simulink model "TST_InjCrv_PoI2AddCor"  (R2016b)
settings: Solver=FixedStepDiscrete  StartTime=0.0  StopTime=simTime  FixedStep=sampleTime  RelTol=1e-3
values from neighbouring files (symbols this model uses):
  testCase = 1    [initTST_InjCrv_PoI2AddCor_001.m]    (also in initTST_InjCrv_PoI2AddCor_002.m = 2; initTST_InjCrv_PoI2AddCor_003.m = 3; initTST_InjCrv_PoI2AddCor_004.m = 4)
libraries: simulink x29, UnitTest_Lib x24
(part 1 of 2)
settings Model: Creator=zhengjinyan  LastModifiedBy=zhengjinyan
settings DebuggingCC: SignalRangeChecking=error

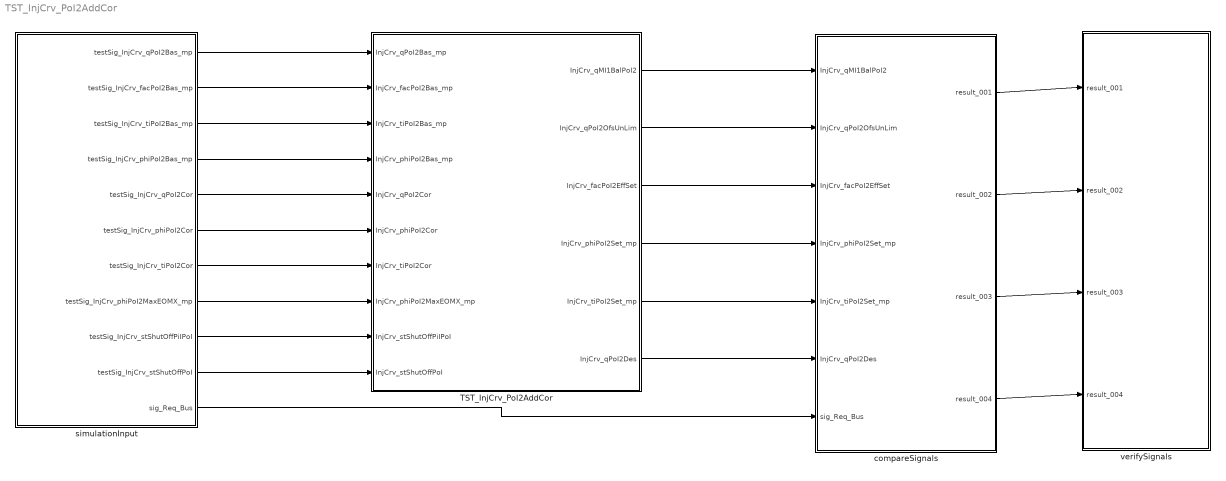
== system TST_InjCrv_PoI2AddCor ==
  TST_InjCrv_PoI2AddCor : Subsystem
  compareSignals : Subsystem
  simulationInput : Subsystem
  verifySignals : Subsystem
  wires:
  simulationInput/1(testSig_InjCrv_qPoI2Bas_mp) -> TST_InjCrv_PoI2AddCor/1(InjCrv_qPoI2Bas_mp)
  simulationInput/2(testSig_InjCrv_facPoI2Bas_mp) -> TST_InjCrv_PoI2AddCor/2(InjCrv_facPoI2Bas_mp)
  simulationInput/3(testSig_InjCrv_tiPoI2Bas_mp) -> TST_InjCrv_PoI2AddCor/3(InjCrv_tiPoI2Bas_mp)
  simulationInput/4(testSig_InjCrv_phiPoI2Bas_mp) -> TST_InjCrv_PoI2AddCor/4(InjCrv_phiPoI2Bas_mp)
  simulationInput/5(testSig_InjCrv_qPoI2Cor) -> TST_InjCrv_PoI2AddCor/5(InjCrv_qPoI2Cor)
  simulationInput/6(testSig_InjCrv_phiPoI2Cor) -> TST_InjCrv_PoI2AddCor/6(InjCrv_phiPoI2Cor)
  simulationInput/7(testSig_InjCrv_tiPoI2Cor) -> TST_InjCrv_PoI2AddCor/7(InjCrv_tiPoI2Cor)
  simulationInput/8(testSig_InjCrv_phiPoI2MaxEOMX_mp) -> TST_InjCrv_PoI2AddCor/8(InjCrv_phiPoI2MaxEOMX_mp)
  simulationInput/9(testSig_InjCrv_stShutOffPiIPoI) -> TST_InjCrv_PoI2AddCor/9(InjCrv_stShutOffPiIPoI)
  simulationInput/10(testSig_InjCrv_stShutOffPoI) -> TST_InjCrv_PoI2AddCor/10(InjCrv_stShutOffPoI)
  TST_InjCrv_PoI2AddCor/1(InjCrv_qMI1BalPoI2) -> compareSignals/1(InjCrv_qMI1BalPoI2)
  TST_InjCrv_PoI2AddCor/2(InjCrv_qPoI2OfsUnLim) -> compareSignals/2(InjCrv_qPoI2OfsUnLim)
  TST_InjCrv_PoI2AddCor/3(InjCrv_facPoI2EffSet) -> compareSignals/3(InjCrv_facPoI2EffSet)
  TST_InjCrv_PoI2AddCor/4(InjCrv_phiPoI2Set_mp) -> compareSignals/4(InjCrv_phiPoI2Set_mp)
  TST_InjCrv_PoI2AddCor/5(InjCrv_tiPoI2Set_mp) -> compareSignals/5(InjCrv_tiPoI2Set_mp)
  TST_InjCrv_PoI2AddCor/6(InjCrv_qPoI2Des) -> compareSignals/6(InjCrv_qPoI2Des)
  simulationInput/11(sig_Req_Bus) -> compareSignals/7(sig_Req_Bus)
  compareSignals/1(result_001) -> verifySignals/1(result_001)
  compareSignals/2(result_002) -> verifySignals/2(result_002)
  compareSignals/3(result_003) -> verifySignals/3(result_003)
  compareSignals/4(result_004) -> verifySignals/4(result_004)

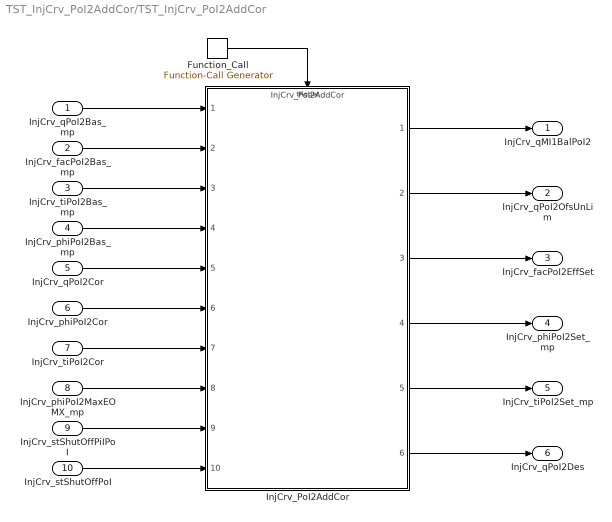
== system TST_InjCrv_PoI2AddCor/TST_InjCrv_PoI2AddCor ==
  InjCrv_qPoI2Bas_mp : Inport
  InjCrv_facPoI2Bas_mp : Inport  Port=2
  InjCrv_tiPoI2Bas_mp : Inport  Port=3
  InjCrv_phiPoI2Bas_mp : Inport  Port=4
  InjCrv_qPoI2Cor : Inport  Port=5
  InjCrv_phiPoI2Cor : Inport  Port=6
  InjCrv_tiPoI2Cor : Inport  Port=7
  InjCrv_phiPoI2MaxEOMX_mp : Inport  Port=8
  InjCrv_stShutOffPiIPoI : Inport  Port=9
  InjCrv_stShutOffPoI : Inport  Port=10
  Function_Call : simulink/Ports & Subsystems/Function-Call Generator  sample_time=sampleTime  numberOfIterations=1
  InjCrv_PoI2AddCor : ModelReference  ModelNameDialog=InjCrv_PoI2AddCor  SimulationMode=Normal  ModelReferenceVersion=1.19  TriggerPortName=function  TriggerPortTriggerType=function-call  TriggerPortStatesWhenEnabling=held
  InjCrv_qMI1BalPoI2 : Outport
  InjCrv_qPoI2OfsUnLim : Outport  Port=2
  InjCrv_facPoI2EffSet : Outport  Port=3
  InjCrv_phiPoI2Set_mp : Outport  Port=4
  InjCrv_tiPoI2Set_mp : Outport  Port=5
  InjCrv_qPoI2Des : Outport  Port=6
  wires:
  Function_Call/1 -> InjCrv_PoI2AddCor/Trigger
  InjCrv_qPoI2Bas_mp/1 -> InjCrv_PoI2AddCor/1
  InjCrv_facPoI2Bas_mp/1 -> InjCrv_PoI2AddCor/2
  InjCrv_tiPoI2Bas_mp/1 -> InjCrv_PoI2AddCor/3
  InjCrv_phiPoI2Bas_mp/1 -> InjCrv_PoI2AddCor/4
  InjCrv_qPoI2Cor/1 -> InjCrv_PoI2AddCor/5
  InjCrv_phiPoI2Cor/1 -> InjCrv_PoI2AddCor/6
  InjCrv_tiPoI2Cor/1 -> InjCrv_PoI2AddCor/7
  InjCrv_phiPoI2MaxEOMX_mp/1 -> InjCrv_PoI2AddCor/8
  InjCrv_stShutOffPiIPoI/1 -> InjCrv_PoI2AddCor/9
  InjCrv_stShutOffPoI/1 -> InjCrv_PoI2AddCor/10
  InjCrv_PoI2AddCor/1 -> InjCrv_qMI1BalPoI2/1
  InjCrv_PoI2AddCor/2 -> InjCrv_qPoI2OfsUnLim/1
  InjCrv_PoI2AddCor/3 -> InjCrv_facPoI2EffSet/1
  InjCrv_PoI2AddCor/4 -> InjCrv_phiPoI2Set_mp/1
  InjCrv_PoI2AddCor/5 -> InjCrv_tiPoI2Set_mp/1
  InjCrv_PoI2AddCor/6 -> InjCrv_qPoI2Des/1

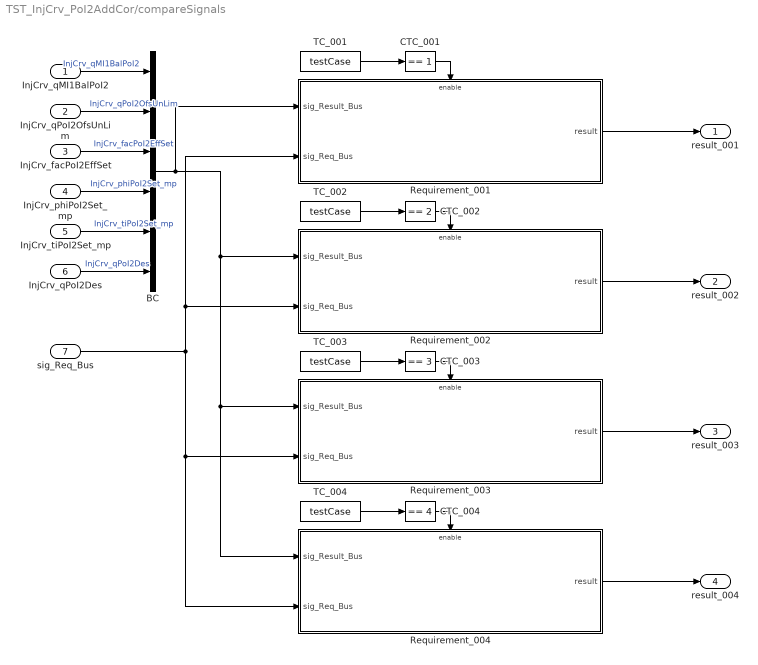
== system TST_InjCrv_PoI2AddCor/compareSignals ==
  InjCrv_qMI1BalPoI2 : Inport
  InjCrv_qPoI2OfsUnLim : Inport  Port=2
  InjCrv_facPoI2EffSet : Inport  Port=3
  InjCrv_phiPoI2Set_mp : Inport  Port=4
  InjCrv_tiPoI2Set_mp : Inport  Port=5
  InjCrv_qPoI2Des : Inport  Port=6
  sig_Req_Bus : Inport  Port=7
  BC : BusCreator  Inputs=6
  CTC_001 : simulink/Logic and Bit Operations/Compare To Constant  relop===  const=1  OutDataTypeStr=boolean
  CTC_002 : simulink/Logic and Bit Operations/Compare To Constant  relop===  const=2  OutDataTypeStr=boolean
  CTC_003 : simulink/Logic and Bit Operations/Compare To Constant  relop===  const=3  OutDataTypeStr=boolean
  CTC_004 : simulink/Logic and Bit Operations/Compare To Constant  relop===  const=4  OutDataTypeStr=boolean
  Requirement_001 : Subsystem
  Requirement_002 : Subsystem
  Requirement_003 : Subsystem
  Requirement_004 : Subsystem
  TC_001 : Constant  Value=testCase
  TC_002 : Constant  Value=testCase
  TC_003 : Constant  Value=testCase
  TC_004 : Constant  Value=testCase
  result_001 : Outport
  result_002 : Outport  Port=2
  result_003 : Outport  Port=3
  result_004 : Outport  Port=4
  wires:
  InjCrv_qMI1BalPoI2/1 -> BC/1  "InjCrv_qMI1BalPoI2"
  InjCrv_qPoI2OfsUnLim/1 -> BC/2  "InjCrv_qPoI2OfsUnLim"
  InjCrv_facPoI2EffSet/1 -> BC/3  "InjCrv_facPoI2EffSet"
  InjCrv_phiPoI2Set_mp/1 -> BC/4  "InjCrv_phiPoI2Set_mp"
  InjCrv_tiPoI2Set_mp/1 -> BC/5  "InjCrv_tiPoI2Set_mp"
  InjCrv_qPoI2Des/1 -> BC/6  "InjCrv_qPoI2Des"
  TC_001/1 -> CTC_001/1
  CTC_001/1 -> Requirement_001/Enable
  sig_Req_Bus/1 -> Requirement_003/2(sig_Req_Bus), Requirement_004/2(sig_Req_Bus), Requirement_001/2(sig_Req_Bus), Requirement_002/2(sig_Req_Bus)
  BC/1 -> Requirement_003/1(sig_Result_Bus), Requirement_004/1(sig_Result_Bus), Requirement_002/1(sig_Result_Bus), Requirement_001/1(sig_Result_Bus)
  Requirement_001/1(result) -> result_001/1
  TC_002/1 -> CTC_002/1
  CTC_002/1 -> Requirement_002/Enable
  Requirement_002/1(result) -> result_002/1
  TC_003/1 -> CTC_003/1
  CTC_003/1 -> Requirement_003/Enable
  Requirement_003/1(result) -> result_003/1
  TC_004/1 -> CTC_004/1
  CTC_004/1 -> Requirement_004/Enable
  Requirement_004/1(result) -> result_004/1

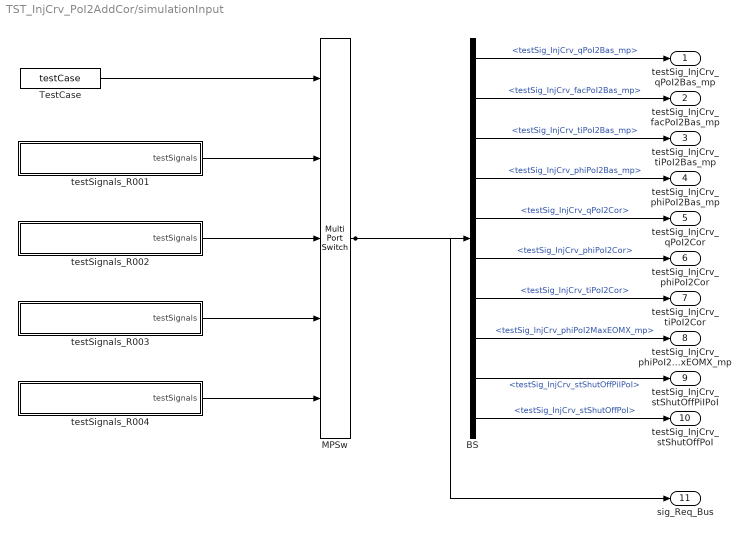
== system TST_InjCrv_PoI2AddCor/simulationInput ==
  BS : BusSelector  OutputSignals=testSig_InjCrv_qPoI2Bas_mp,testSig_InjCrv_facPoI2Bas_mp,testSig_InjCrv_tiPoI2Bas_mp,testSig_InjCrv_phiPoI2Bas_mp,testSig_InjCrv_qPoI2Cor,testSig_InjCrv_phiPoI2Cor,testSig_InjCrv_tiPoI2Cor,testSig_InjCrv_phiPoI2MaxEOMX_mp,testSig_InjCrv_stShutOffPiIPoI,testSig_InjCrv_stShutOffPoI
  MPSw : MultiPortSwitch  Inputs=4  SaturateOnIntegerOverflow=on  InputSameDT=on
  TestCase : Constant  Value=testCase
  testSignals_R001 : Subsystem
  testSignals_R002 : Subsystem
  testSignals_R003 : Subsystem
  testSignals_R004 : Subsystem
  testSig_InjCrv_qPoI2Bas_mp : Outport
  testSig_InjCrv_facPoI2Bas_mp : Outport  Port=2
  testSig_InjCrv_tiPoI2Bas_mp : Outport  Port=3
  testSig_InjCrv_phiPoI2Bas_mp : Outport  Port=4
  testSig_InjCrv_qPoI2Cor : Outport  Port=5
  testSig_InjCrv_phiPoI2Cor : Outport  Port=6
  testSig_InjCrv_tiPoI2Cor : Outport  Port=7
  testSig_InjCrv_phiPoI2MaxEOMX_mp : Outport  Port=8
  testSig_InjCrv_stShutOffPiIPoI : Outport  Port=9
  testSig_InjCrv_stShutOffPoI : Outport  Port=10
  sig_Req_Bus : Outport  Port=11
  wires:
  BS/1 -> testSig_InjCrv_qPoI2Bas_mp/1  "<testSig_InjCrv_qPoI2Bas_mp>"
  BS/2 -> testSig_InjCrv_facPoI2Bas_mp/1  "<testSig_InjCrv_facPoI2Bas_mp>"
  BS/3 -> testSig_InjCrv_tiPoI2Bas_mp/1  "<testSig_InjCrv_tiPoI2Bas_mp>"
  BS/4 -> testSig_InjCrv_phiPoI2Bas_mp/1  "<testSig_InjCrv_phiPoI2Bas_mp>"
  BS/5 -> testSig_InjCrv_qPoI2Cor/1  "<testSig_InjCrv_qPoI2Cor>"
  BS/6 -> testSig_InjCrv_phiPoI2Cor/1  "<testSig_InjCrv_phiPoI2Cor>"
  BS/7 -> testSig_InjCrv_tiPoI2Cor/1  "<testSig_InjCrv_tiPoI2Cor>"
  BS/8 -> testSig_InjCrv_phiPoI2MaxEOMX_mp/1  "<testSig_InjCrv_phiPoI2MaxEOMX_mp>"
  BS/9 -> testSig_InjCrv_stShutOffPiIPoI/1  "<testSig_InjCrv_stShutOffPiIPoI>"
  BS/10 -> testSig_InjCrv_stShutOffPoI/1  "<testSig_InjCrv_stShutOffPoI>"
  MPSw/1 -> BS/1, sig_Req_Bus/1
  TestCase/1 -> MPSw/1
  testSignals_R001/1(testSignals) -> MPSw/2
  testSignals_R002/1(testSignals) -> MPSw/3
  testSignals_R003/1(testSignals) -> MPSw/4
  testSignals_R004/1(testSignals) -> MPSw/5

== system TST_InjCrv_PoI2AddCor/verifySignals ==
  result_001 : Inport
  result_002 : Inport  Port=2
  result_003 : Inport  Port=3
  result_004 : Inport  Port=4
  Assertion_001 : Assertion  Enabled=off
  Assertion_002 : Assertion  Enabled=off
  Assertion_003 : Assertion  Enabled=off
  Assertion_004 : Assertion  Enabled=off
  wires:
  result_001/1 -> Assertion_001/1
  result_002/1 -> Assertion_002/1
  result_003/1 -> Assertion_003/1
  result_004/1 -> Assertion_004/1

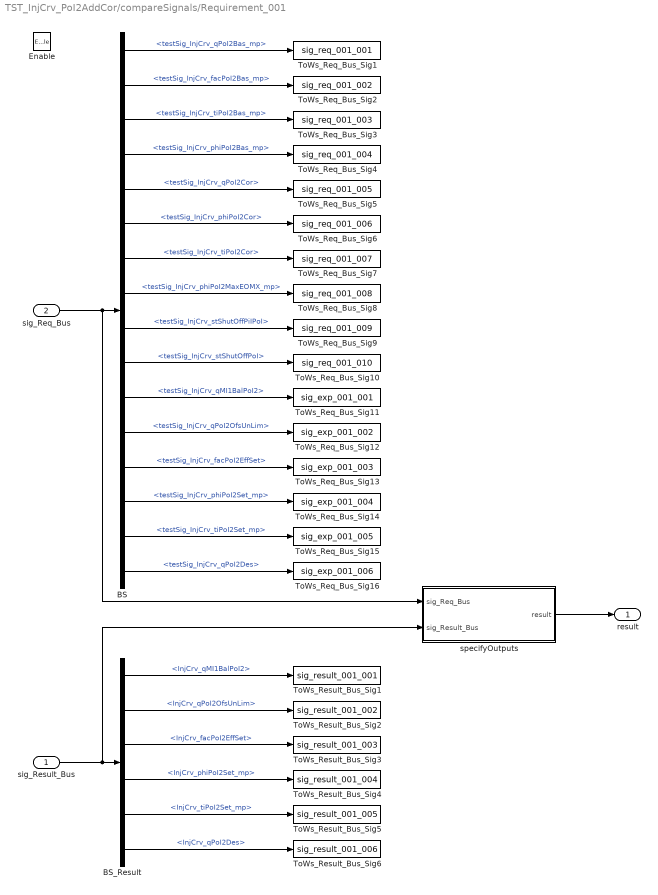
== system TST_InjCrv_PoI2AddCor/compareSignals/Requirement_001 ==
  sig_Result_Bus : Inport
  sig_Req_Bus : Inport  Port=2
  Enable : EnablePort
  BS : BusSelector  OutputSignals=testSig_InjCrv_qPoI2Bas_mp,testSig_InjCrv_facPoI2Bas_mp,testSig_InjCrv_tiPoI2Bas_mp,testSig_InjCrv_phiPoI2Bas_mp,testSig_InjCrv_qPoI2Cor,testSig_InjCrv_phiPoI2Cor,testSig_InjCrv_tiPoI2Cor,testSig_InjCrv_phiPoI2MaxEOMX_mp,testSig_InjCrv_stShutOffPiIPoI,testSig_InjCrv_stShutOffPoI,testSig_InjCrv_qMI1BalPoI2,testSig_InjCrv_qPoI2OfsUnLim,testSig_InjCrv_facPoI2EffSet,testSig_InjCrv_phiPoI2Set_mp,testSig_InjCrv_tiPoI2Set_mp,testSig_InjCrv_qPoI2Des
  BS_Result : BusSelector  OutputSignals=InjCrv_qMI1BalPoI2,InjCrv_qPoI2OfsUnLim,InjCrv_facPoI2EffSet,InjCrv_phiPoI2Set_mp,InjCrv_tiPoI2Set_mp,InjCrv_qPoI2Des
  ToWs_Req_Bus_Sig1 : ToWorkspace  VariableName=sig_req_001_001  SaveFormat=Structure With Time
  ToWs_Req_Bus_Sig10 : ToWorkspace  VariableName=sig_req_001_010  SaveFormat=Structure With Time
  ToWs_Req_Bus_Sig11 : ToWorkspace  VariableName=sig_exp_001_001  SaveFormat=Structure With Time
  ToWs_Req_Bus_Sig12 : ToWorkspace  VariableName=sig_exp_001_002  SaveFormat=Structure With Time
  ToWs_Req_Bus_Sig13 : ToWorkspace  VariableName=sig_exp_001_003  SaveFormat=Structure With Time
  ToWs_Req_Bus_Sig14 : ToWorkspace  VariableName=sig_exp_001_004  SaveFormat=Structure With Time
  ToWs_Req_Bus_Sig15 : ToWorkspace  VariableName=sig_exp_001_005  SaveFormat=Structure With Time
  ToWs_Req_Bus_Sig16 : ToWorkspace  VariableName=sig_exp_001_006  SaveFormat=Structure With Time
  ToWs_Req_Bus_Sig2 : ToWorkspace  VariableName=sig_req_001_002  SaveFormat=Structure With Time
  ToWs_Req_Bus_Sig3 : ToWorkspace  VariableName=sig_req_001_003  SaveFormat=Structure With Time
  ToWs_Req_Bus_Sig4 : ToWorkspace  VariableName=sig_req_001_004  SaveFormat=Structure With Time
  ToWs_Req_Bus_Sig5 : ToWorkspace  VariableName=sig_req_001_005  SaveFormat=Structure With Time
  ToWs_Req_Bus_Sig6 : ToWorkspace  VariableName=sig_req_001_006  SaveFormat=Structure With Time
  ToWs_Req_Bus_Sig7 : ToWorkspace  VariableName=sig_req_001_007  SaveFormat=Structure With Time
  ToWs_Req_Bus_Sig8 : ToWorkspace  VariableName=sig_req_001_008  SaveFormat=Structure With Time
  ToWs_Req_Bus_Sig9 : ToWorkspace  VariableName=sig_req_001_009  SaveFormat=Structure With Time
  ToWs_Result_Bus_Sig1 : ToWorkspace  VariableName=sig_result_001_001  SaveFormat=Structure With Time
  ToWs_Result_Bus_Sig2 : ToWorkspace  VariableName=sig_result_001_002  SaveFormat=Structure With Time
  ToWs_Result_Bus_Sig3 : ToWorkspace  VariableName=sig_result_001_003  SaveFormat=Structure With Time
  ToWs_Result_Bus_Sig4 : ToWorkspace  VariableName=sig_result_001_004  SaveFormat=Structure With Time
  ToWs_Result_Bus_Sig5 : ToWorkspace  VariableName=sig_result_001_005  SaveFormat=Structure With Time
  ToWs_Result_Bus_Sig6 : ToWorkspace  VariableName=sig_result_001_006  SaveFormat=Structure With Time
  specifyOutputs : Subsystem
  result : Outport
  wires:
  sig_Req_Bus/1 -> BS/1, specifyOutputs/1(sig_Req_Bus)
  BS/1 -> ToWs_Req_Bus_Sig1/1  "<testSig_InjCrv_qPoI2Bas_mp>"
  BS/2 -> ToWs_Req_Bus_Sig2/1  "<testSig_InjCrv_facPoI2Bas_mp>"
  BS/3 -> ToWs_Req_Bus_Sig3/1  "<testSig_InjCrv_tiPoI2Bas_mp>"
  BS/4 -> ToWs_Req_Bus_Sig4/1  "<testSig_InjCrv_phiPoI2Bas_mp>"
  BS/5 -> ToWs_Req_Bus_Sig5/1  "<testSig_InjCrv_qPoI2Cor>"
  BS/6 -> ToWs_Req_Bus_Sig6/1  "<testSig_InjCrv_phiPoI2Cor>"
  BS/7 -> ToWs_Req_Bus_Sig7/1  "<testSig_InjCrv_tiPoI2Cor>"
  BS/8 -> ToWs_Req_Bus_Sig8/1  "<testSig_InjCrv_phiPoI2MaxEOMX_mp>"
  BS/9 -> ToWs_Req_Bus_Sig9/1  "<testSig_InjCrv_stShutOffPiIPoI>"
  BS/10 -> ToWs_Req_Bus_Sig10/1  "<testSig_InjCrv_stShutOffPoI>"
  BS/11 -> ToWs_Req_Bus_Sig11/1  "<testSig_InjCrv_qMI1BalPoI2>"
  BS/12 -> ToWs_Req_Bus_Sig12/1  "<testSig_InjCrv_qPoI2OfsUnLim>"
  BS/13 -> ToWs_Req_Bus_Sig13/1  "<testSig_InjCrv_facPoI2EffSet>"
  BS/14 -> ToWs_Req_Bus_Sig14/1  "<testSig_InjCrv_phiPoI2Set_mp>"
  BS/15 -> ToWs_Req_Bus_Sig15/1  "<testSig_InjCrv_tiPoI2Set_mp>"
  BS/16 -> ToWs_Req_Bus_Sig16/1  "<testSig_InjCrv_qPoI2Des>"
  sig_Result_Bus/1 -> BS_Result/1, specifyOutputs/2(sig_Result_Bus)
  BS_Result/1 -> ToWs_Result_Bus_Sig1/1  "<InjCrv_qMI1BalPoI2>"
  BS_Result/2 -> ToWs_Result_Bus_Sig2/1  "<InjCrv_qPoI2OfsUnLim>"
  BS_Result/3 -> ToWs_Result_Bus_Sig3/1  "<InjCrv_facPoI2EffSet>"
  BS_Result/4 -> ToWs_Result_Bus_Sig4/1  "<InjCrv_phiPoI2Set_mp>"
  BS_Result/5 -> ToWs_Result_Bus_Sig5/1  "<InjCrv_tiPoI2Set_mp>"
  BS_Result/6 -> ToWs_Result_Bus_Sig6/1  "<InjCrv_qPoI2Des>"
  specifyOutputs/1(result) -> result/1

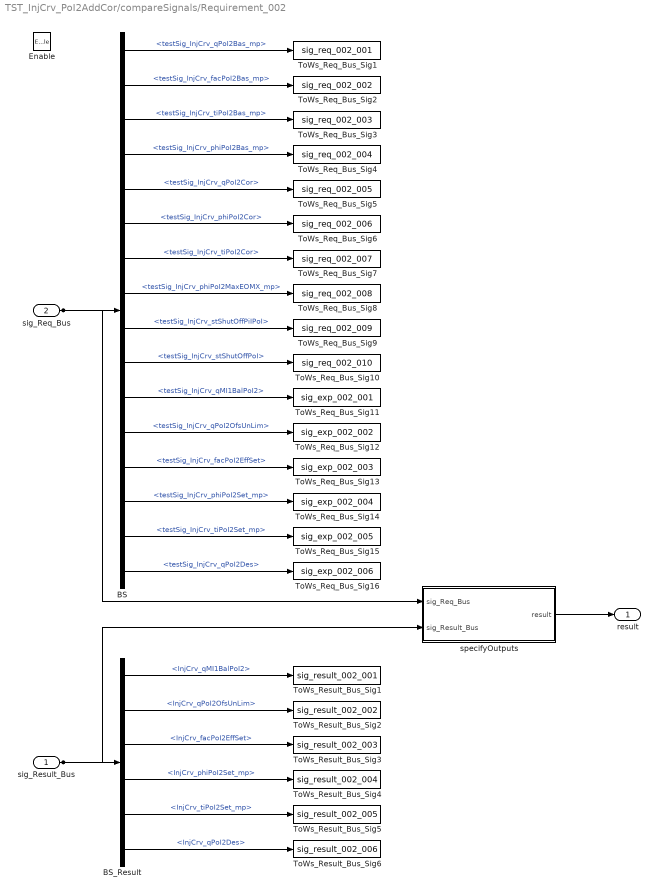
== system TST_InjCrv_PoI2AddCor/compareSignals/Requirement_002 ==
  sig_Result_Bus : Inport
  sig_Req_Bus : Inport  Port=2
  Enable : EnablePort
  BS : BusSelector  OutputSignals=testSig_InjCrv_qPoI2Bas_mp,testSig_InjCrv_facPoI2Bas_mp,testSig_InjCrv_tiPoI2Bas_mp,testSig_InjCrv_phiPoI2Bas_mp,testSig_InjCrv_qPoI2Cor,testSig_InjCrv_phiPoI2Cor,testSig_InjCrv_tiPoI2Cor,testSig_InjCrv_phiPoI2MaxEOMX_mp,testSig_InjCrv_stShutOffPiIPoI,testSig_InjCrv_stShutOffPoI,testSig_InjCrv_qMI1BalPoI2,testSig_InjCrv_qPoI2OfsUnLim,testSig_InjCrv_facPoI2EffSet,testSig_InjCrv_phiPoI2Set_mp,testSig_InjCrv_tiPoI2Set_mp,testSig_InjCrv_qPoI2Des
  BS_Result : BusSelector  OutputSignals=InjCrv_qMI1BalPoI2,InjCrv_qPoI2OfsUnLim,InjCrv_facPoI2EffSet,InjCrv_phiPoI2Set_mp,InjCrv_tiPoI2Set_mp,InjCrv_qPoI2Des
  ToWs_Req_Bus_Sig1 : ToWorkspace  VariableName=sig_req_002_001  SaveFormat=Structure With Time
  ToWs_Req_Bus_Sig10 : ToWorkspace  VariableName=sig_req_002_010  SaveFormat=Structure With Time
  ToWs_Req_Bus_Sig11 : ToWorkspace  VariableName=sig_exp_002_001  SaveFormat=Structure With Time
  ToWs_Req_Bus_Sig12 : ToWorkspace  VariableName=sig_exp_002_002  SaveFormat=Structure With Time
  ToWs_Req_Bus_Sig13 : ToWorkspace  VariableName=sig_exp_002_003  SaveFormat=Structure With Time
  ToWs_Req_Bus_Sig14 : ToWorkspace  VariableName=sig_exp_002_004  SaveFormat=Structure With Time
  ToWs_Req_Bus_Sig15 : ToWorkspace  VariableName=sig_exp_002_005  SaveFormat=Structure With Time
  ToWs_Req_Bus_Sig16 : ToWorkspace  VariableName=sig_exp_002_006  SaveFormat=Structure With Time
  ToWs_Req_Bus_Sig2 : ToWorkspace  VariableName=sig_req_002_002  SaveFormat=Structure With Time
  ToWs_Req_Bus_Sig3 : ToWorkspace  VariableName=sig_req_002_003  SaveFormat=Structure With Time
  ToWs_Req_Bus_Sig4 : ToWorkspace  VariableName=sig_req_002_004  SaveFormat=Structure With Time
  ToWs_Req_Bus_Sig5 : ToWorkspace  VariableName=sig_req_002_005  SaveFormat=Structure With Time
  ToWs_Req_Bus_Sig6 : ToWorkspace  VariableName=sig_req_002_006  SaveFormat=Structure With Time
  ToWs_Req_Bus_Sig7 : ToWorkspace  VariableName=sig_req_002_007  SaveFormat=Structure With Time
  ToWs_Req_Bus_Sig8 : ToWorkspace  VariableName=sig_req_002_008  SaveFormat=Structure With Time
  ToWs_Req_Bus_Sig9 : ToWorkspace  VariableName=sig_req_002_009  SaveFormat=Structure With Time
  ToWs_Result_Bus_Sig1 : ToWorkspace  VariableName=sig_result_002_001  SaveFormat=Structure With Time
  ToWs_Result_Bus_Sig2 : ToWorkspace  VariableName=sig_result_002_002  SaveFormat=Structure With Time
  ToWs_Result_Bus_Sig3 : ToWorkspace  VariableName=sig_result_002_003  SaveFormat=Structure With Time
  ToWs_Result_Bus_Sig4 : ToWorkspace  VariableName=sig_result_002_004  SaveFormat=Structure With Time
  ToWs_Result_Bus_Sig5 : ToWorkspace  VariableName=sig_result_002_005  SaveFormat=Structure With Time
  ToWs_Result_Bus_Sig6 : ToWorkspace  VariableName=sig_result_002_006  SaveFormat=Structure With Time
  specifyOutputs : Subsystem
  result : Outport
  wires:
  sig_Req_Bus/1 -> BS/1, specifyOutputs/1(sig_Req_Bus)
  BS/1 -> ToWs_Req_Bus_Sig1/1  "<testSig_InjCrv_qPoI2Bas_mp>"
  BS/2 -> ToWs_Req_Bus_Sig2/1  "<testSig_InjCrv_facPoI2Bas_mp>"
  BS/3 -> ToWs_Req_Bus_Sig3/1  "<testSig_InjCrv_tiPoI2Bas_mp>"
  BS/4 -> ToWs_Req_Bus_Sig4/1  "<testSig_InjCrv_phiPoI2Bas_mp>"
  BS/5 -> ToWs_Req_Bus_Sig5/1  "<testSig_InjCrv_qPoI2Cor>"
  BS/6 -> ToWs_Req_Bus_Sig6/1  "<testSig_InjCrv_phiPoI2Cor>"
  BS/7 -> ToWs_Req_Bus_Sig7/1  "<testSig_InjCrv_tiPoI2Cor>"
  BS/8 -> ToWs_Req_Bus_Sig8/1  "<testSig_InjCrv_phiPoI2MaxEOMX_mp>"
  BS/9 -> ToWs_Req_Bus_Sig9/1  "<testSig_InjCrv_stShutOffPiIPoI>"
  BS/10 -> ToWs_Req_Bus_Sig10/1  "<testSig_InjCrv_stShutOffPoI>"
  BS/11 -> ToWs_Req_Bus_Sig11/1  "<testSig_InjCrv_qMI1BalPoI2>"
  BS/12 -> ToWs_Req_Bus_Sig12/1  "<testSig_InjCrv_qPoI2OfsUnLim>"
  BS/13 -> ToWs_Req_Bus_Sig13/1  "<testSig_InjCrv_facPoI2EffSet>"
  BS/14 -> ToWs_Req_Bus_Sig14/1  "<testSig_InjCrv_phiPoI2Set_mp>"
  BS/15 -> ToWs_Req_Bus_Sig15/1  "<testSig_InjCrv_tiPoI2Set_mp>"
  BS/16 -> ToWs_Req_Bus_Sig16/1  "<testSig_InjCrv_qPoI2Des>"
  sig_Result_Bus/1 -> BS_Result/1, specifyOutputs/2(sig_Result_Bus)
  BS_Result/1 -> ToWs_Result_Bus_Sig1/1  "<InjCrv_qMI1BalPoI2>"
  BS_Result/2 -> ToWs_Result_Bus_Sig2/1  "<InjCrv_qPoI2OfsUnLim>"
  BS_Result/3 -> ToWs_Result_Bus_Sig3/1  "<InjCrv_facPoI2EffSet>"
  BS_Result/4 -> ToWs_Result_Bus_Sig4/1  "<InjCrv_phiPoI2Set_mp>"
  BS_Result/5 -> ToWs_Result_Bus_Sig5/1  "<InjCrv_tiPoI2Set_mp>"
  BS_Result/6 -> ToWs_Result_Bus_Sig6/1  "<InjCrv_qPoI2Des>"
  specifyOutputs/1(result) -> result/1

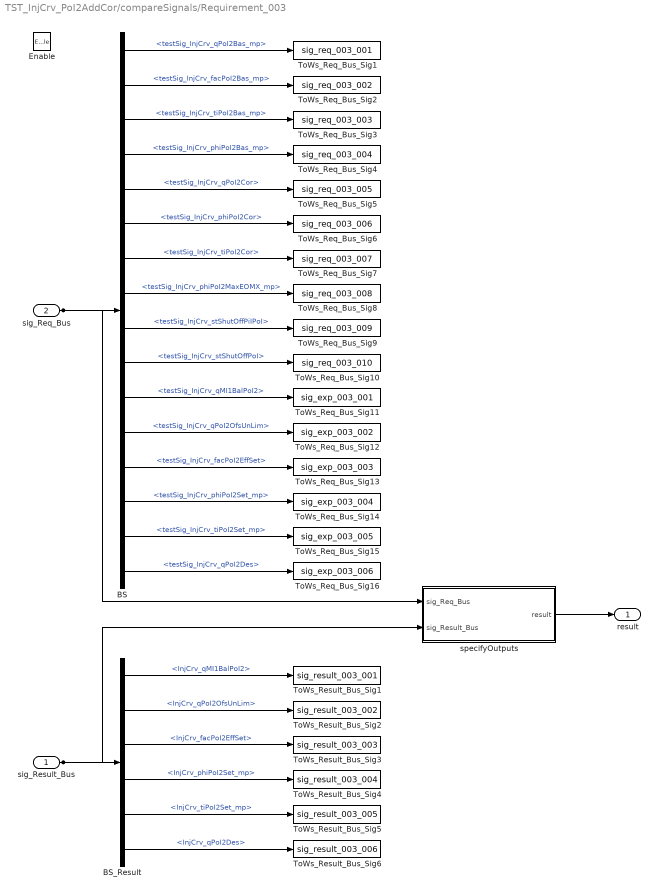
== system TST_InjCrv_PoI2AddCor/compareSignals/Requirement_003 ==
  sig_Result_Bus : Inport
  sig_Req_Bus : Inport  Port=2
  Enable : EnablePort
  BS : BusSelector  OutputSignals=testSig_InjCrv_qPoI2Bas_mp,testSig_InjCrv_facPoI2Bas_mp,testSig_InjCrv_tiPoI2Bas_mp,testSig_InjCrv_phiPoI2Bas_mp,testSig_InjCrv_qPoI2Cor,testSig_InjCrv_phiPoI2Cor,testSig_InjCrv_tiPoI2Cor,testSig_InjCrv_phiPoI2MaxEOMX_mp,testSig_InjCrv_stShutOffPiIPoI,testSig_InjCrv_stShutOffPoI,testSig_InjCrv_qMI1BalPoI2,testSig_InjCrv_qPoI2OfsUnLim,testSig_InjCrv_facPoI2EffSet,testSig_InjCrv_phiPoI2Set_mp,testSig_InjCrv_tiPoI2Set_mp,testSig_InjCrv_qPoI2Des
  BS_Result : BusSelector  OutputSignals=InjCrv_qMI1BalPoI2,InjCrv_qPoI2OfsUnLim,InjCrv_facPoI2EffSet,InjCrv_phiPoI2Set_mp,InjCrv_tiPoI2Set_mp,InjCrv_qPoI2Des
  ToWs_Req_Bus_Sig1 : ToWorkspace  VariableName=sig_req_003_001  SaveFormat=Structure With Time
  ToWs_Req_Bus_Sig10 : ToWorkspace  VariableName=sig_req_003_010  SaveFormat=Structure With Time
  ToWs_Req_Bus_Sig11 : ToWorkspace  VariableName=sig_exp_003_001  SaveFormat=Structure With Time
  ToWs_Req_Bus_Sig12 : ToWorkspace  VariableName=sig_exp_003_002  SaveFormat=Structure With Time
  ToWs_Req_Bus_Sig13 : ToWorkspace  VariableName=sig_exp_003_003  SaveFormat=Structure With Time
  ToWs_Req_Bus_Sig14 : ToWorkspace  VariableName=sig_exp_003_004  SaveFormat=Structure With Time
  ToWs_Req_Bus_Sig15 : ToWorkspace  VariableName=sig_exp_003_005  SaveFormat=Structure With Time
  ToWs_Req_Bus_Sig16 : ToWorkspace  VariableName=sig_exp_003_006  SaveFormat=Structure With Time
  ToWs_Req_Bus_Sig2 : ToWorkspace  VariableName=sig_req_003_002  SaveFormat=Structure With Time
  ToWs_Req_Bus_Sig3 : ToWorkspace  VariableName=sig_req_003_003  SaveFormat=Structure With Time
  ToWs_Req_Bus_Sig4 : ToWorkspace  VariableName=sig_req_003_004  SaveFormat=Structure With Time
  ToWs_Req_Bus_Sig5 : ToWorkspace  VariableName=sig_req_003_005  SaveFormat=Structure With Time
  ToWs_Req_Bus_Sig6 : ToWorkspace  VariableName=sig_req_003_006  SaveFormat=Structure With Time
  ToWs_Req_Bus_Sig7 : ToWorkspace  VariableName=sig_req_003_007  SaveFormat=Structure With Time
  ToWs_Req_Bus_Sig8 : ToWorkspace  VariableName=sig_req_003_008  SaveFormat=Structure With Time
  ToWs_Req_Bus_Sig9 : ToWorkspace  VariableName=sig_req_003_009  SaveFormat=Structure With Time
  ToWs_Result_Bus_Sig1 : ToWorkspace  VariableName=sig_result_003_001  SaveFormat=Structure With Time
  ToWs_Result_Bus_Sig2 : ToWorkspace  VariableName=sig_result_003_002  SaveFormat=Structure With Time
  ToWs_Result_Bus_Sig3 : ToWorkspace  VariableName=sig_result_003_003  SaveFormat=Structure With Time
  ToWs_Result_Bus_Sig4 : ToWorkspace  VariableName=sig_result_003_004  SaveFormat=Structure With Time
  ToWs_Result_Bus_Sig5 : ToWorkspace  VariableName=sig_result_003_005  SaveFormat=Structure With Time
  ToWs_Result_Bus_Sig6 : ToWorkspace  VariableName=sig_result_003_006  SaveFormat=Structure With Time
  specifyOutputs : Subsystem
  result : Outport
  wires:
  sig_Req_Bus/1 -> BS/1, specifyOutputs/1(sig_Req_Bus)
  BS/1 -> ToWs_Req_Bus_Sig1/1  "<testSig_InjCrv_qPoI2Bas_mp>"
  BS/2 -> ToWs_Req_Bus_Sig2/1  "<testSig_InjCrv_facPoI2Bas_mp>"
  BS/3 -> ToWs_Req_Bus_Sig3/1  "<testSig_InjCrv_tiPoI2Bas_mp>"
  BS/4 -> ToWs_Req_Bus_Sig4/1  "<testSig_InjCrv_phiPoI2Bas_mp>"
  BS/5 -> ToWs_Req_Bus_Sig5/1  "<testSig_InjCrv_qPoI2Cor>"
  BS/6 -> ToWs_Req_Bus_Sig6/1  "<testSig_InjCrv_phiPoI2Cor>"
  BS/7 -> ToWs_Req_Bus_Sig7/1  "<testSig_InjCrv_tiPoI2Cor>"
  BS/8 -> ToWs_Req_Bus_Sig8/1  "<testSig_InjCrv_phiPoI2MaxEOMX_mp>"
  BS/9 -> ToWs_Req_Bus_Sig9/1  "<testSig_InjCrv_stShutOffPiIPoI>"
  BS/10 -> ToWs_Req_Bus_Sig10/1  "<testSig_InjCrv_stShutOffPoI>"
  BS/11 -> ToWs_Req_Bus_Sig11/1  "<testSig_InjCrv_qMI1BalPoI2>"
  BS/12 -> ToWs_Req_Bus_Sig12/1  "<testSig_InjCrv_qPoI2OfsUnLim>"
  BS/13 -> ToWs_Req_Bus_Sig13/1  "<testSig_InjCrv_facPoI2EffSet>"
  BS/14 -> ToWs_Req_Bus_Sig14/1  "<testSig_InjCrv_phiPoI2Set_mp>"
  BS/15 -> ToWs_Req_Bus_Sig15/1  "<testSig_InjCrv_tiPoI2Set_mp>"
  BS/16 -> ToWs_Req_Bus_Sig16/1  "<testSig_InjCrv_qPoI2Des>"
  sig_Result_Bus/1 -> BS_Result/1, specifyOutputs/2(sig_Result_Bus)
  BS_Result/1 -> ToWs_Result_Bus_Sig1/1  "<InjCrv_qMI1BalPoI2>"
  BS_Result/2 -> ToWs_Result_Bus_Sig2/1  "<InjCrv_qPoI2OfsUnLim>"
  BS_Result/3 -> ToWs_Result_Bus_Sig3/1  "<InjCrv_facPoI2EffSet>"
  BS_Result/4 -> ToWs_Result_Bus_Sig4/1  "<InjCrv_phiPoI2Set_mp>"
  BS_Result/5 -> ToWs_Result_Bus_Sig5/1  "<InjCrv_tiPoI2Set_mp>"
  BS_Result/6 -> ToWs_Result_Bus_Sig6/1  "<InjCrv_qPoI2Des>"
  specifyOutputs/1(result) -> result/1

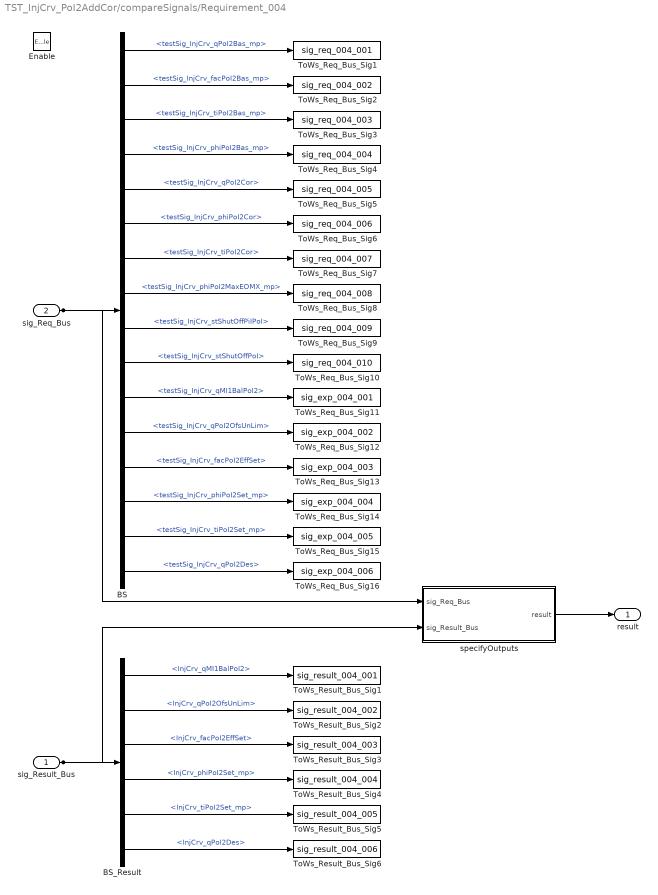
== system TST_InjCrv_PoI2AddCor/compareSignals/Requirement_004 ==
  sig_Result_Bus : Inport
  sig_Req_Bus : Inport  Port=2
  Enable : EnablePort
  BS : BusSelector  OutputSignals=testSig_InjCrv_qPoI2Bas_mp,testSig_InjCrv_facPoI2Bas_mp,testSig_InjCrv_tiPoI2Bas_mp,testSig_InjCrv_phiPoI2Bas_mp,testSig_InjCrv_qPoI2Cor,testSig_InjCrv_phiPoI2Cor,testSig_InjCrv_tiPoI2Cor,testSig_InjCrv_phiPoI2MaxEOMX_mp,testSig_InjCrv_stShutOffPiIPoI,testSig_InjCrv_stShutOffPoI,testSig_InjCrv_qMI1BalPoI2,testSig_InjCrv_qPoI2OfsUnLim,testSig_InjCrv_facPoI2EffSet,testSig_InjCrv_phiPoI2Set_mp,testSig_InjCrv_tiPoI2Set_mp,testSig_InjCrv_qPoI2Des
  BS_Result : BusSelector  OutputSignals=InjCrv_qMI1BalPoI2,InjCrv_qPoI2OfsUnLim,InjCrv_facPoI2EffSet,InjCrv_phiPoI2Set_mp,InjCrv_tiPoI2Set_mp,InjCrv_qPoI2Des
  ToWs_Req_Bus_Sig1 : ToWorkspace  VariableName=sig_req_004_001  SaveFormat=Structure With Time
  ToWs_Req_Bus_Sig10 : ToWorkspace  VariableName=sig_req_004_010  SaveFormat=Structure With Time
  ToWs_Req_Bus_Sig11 : ToWorkspace  VariableName=sig_exp_004_001  SaveFormat=Structure With Time
  ToWs_Req_Bus_Sig12 : ToWorkspace  VariableName=sig_exp_004_002  SaveFormat=Structure With Time
  ToWs_Req_Bus_Sig13 : ToWorkspace  VariableName=sig_exp_004_003  SaveFormat=Structure With Time
  ToWs_Req_Bus_Sig14 : ToWorkspace  VariableName=sig_exp_004_004  SaveFormat=Structure With Time
  ToWs_Req_Bus_Sig15 : ToWorkspace  VariableName=sig_exp_004_005  SaveFormat=Structure With Time
  ToWs_Req_Bus_Sig16 : ToWorkspace  VariableName=sig_exp_004_006  SaveFormat=Structure With Time
  ToWs_Req_Bus_Sig2 : ToWorkspace  VariableName=sig_req_004_002  SaveFormat=Structure With Time
  ToWs_Req_Bus_Sig3 : ToWorkspace  VariableName=sig_req_004_003  SaveFormat=Structure With Time
  ToWs_Req_Bus_Sig4 : ToWorkspace  VariableName=sig_req_004_004  SaveFormat=Structure With Time
  ToWs_Req_Bus_Sig5 : ToWorkspace  VariableName=sig_req_004_005  SaveFormat=Structure With Time
  ToWs_Req_Bus_Sig6 : ToWorkspace  VariableName=sig_req_004_006  SaveFormat=Structure With Time
  ToWs_Req_Bus_Sig7 : ToWorkspace  VariableName=sig_req_004_007  SaveFormat=Structure With Time
  ToWs_Req_Bus_Sig8 : ToWorkspace  VariableName=sig_req_004_008  SaveFormat=Structure With Time
  ToWs_Req_Bus_Sig9 : ToWorkspace  VariableName=sig_req_004_009  SaveFormat=Structure With Time
  ToWs_Result_Bus_Sig1 : ToWorkspace  VariableName=sig_result_004_001  SaveFormat=Structure With Time
  ToWs_Result_Bus_Sig2 : ToWorkspace  VariableName=sig_result_004_002  SaveFormat=Structure With Time
  ToWs_Result_Bus_Sig3 : ToWorkspace  VariableName=sig_result_004_003  SaveFormat=Structure With Time
  ToWs_Result_Bus_Sig4 : ToWorkspace  VariableName=sig_result_004_004  SaveFormat=Structure With Time
  ToWs_Result_Bus_Sig5 : ToWorkspace  VariableName=sig_result_004_005  SaveFormat=Structure With Time
  ToWs_Result_Bus_Sig6 : ToWorkspace  VariableName=sig_result_004_006  SaveFormat=Structure With Time
  specifyOutputs : Subsystem
  result : Outport
  wires:
  sig_Req_Bus/1 -> BS/1, specifyOutputs/1(sig_Req_Bus)
  BS/1 -> ToWs_Req_Bus_Sig1/1  "<testSig_InjCrv_qPoI2Bas_mp>"
  BS/2 -> ToWs_Req_Bus_Sig2/1  "<testSig_InjCrv_facPoI2Bas_mp>"
  BS/3 -> ToWs_Req_Bus_Sig3/1  "<testSig_InjCrv_tiPoI2Bas_mp>"
  BS/4 -> ToWs_Req_Bus_Sig4/1  "<testSig_InjCrv_phiPoI2Bas_mp>"
  BS/5 -> ToWs_Req_Bus_Sig5/1  "<testSig_InjCrv_qPoI2Cor>"
  BS/6 -> ToWs_Req_Bus_Sig6/1  "<testSig_InjCrv_phiPoI2Cor>"
  BS/7 -> ToWs_Req_Bus_Sig7/1  "<testSig_InjCrv_tiPoI2Cor>"
  BS/8 -> ToWs_Req_Bus_Sig8/1  "<testSig_InjCrv_phiPoI2MaxEOMX_mp>"
  BS/9 -> ToWs_Req_Bus_Sig9/1  "<testSig_InjCrv_stShutOffPiIPoI>"
  BS/10 -> ToWs_Req_Bus_Sig10/1  "<testSig_InjCrv_stShutOffPoI>"
  BS/11 -> ToWs_Req_Bus_Sig11/1  "<testSig_InjCrv_qMI1BalPoI2>"
  BS/12 -> ToWs_Req_Bus_Sig12/1  "<testSig_InjCrv_qPoI2OfsUnLim>"
  BS/13 -> ToWs_Req_Bus_Sig13/1  "<testSig_InjCrv_facPoI2EffSet>"
  BS/14 -> ToWs_Req_Bus_Sig14/1  "<testSig_InjCrv_phiPoI2Set_mp>"
  BS/15 -> ToWs_Req_Bus_Sig15/1  "<testSig_InjCrv_tiPoI2Set_mp>"
  BS/16 -> ToWs_Req_Bus_Sig16/1  "<testSig_InjCrv_qPoI2Des>"
  sig_Result_Bus/1 -> BS_Result/1, specifyOutputs/2(sig_Result_Bus)
  BS_Result/1 -> ToWs_Result_Bus_Sig1/1  "<InjCrv_qMI1BalPoI2>"
  BS_Result/2 -> ToWs_Result_Bus_Sig2/1  "<InjCrv_qPoI2OfsUnLim>"
  BS_Result/3 -> ToWs_Result_Bus_Sig3/1  "<InjCrv_facPoI2EffSet>"
  BS_Result/4 -> ToWs_Result_Bus_Sig4/1  "<InjCrv_phiPoI2Set_mp>"
  BS_Result/5 -> ToWs_Result_Bus_Sig5/1  "<InjCrv_tiPoI2Set_mp>"
  BS_Result/6 -> ToWs_Result_Bus_Sig6/1  "<InjCrv_qPoI2Des>"
  specifyOutputs/1(result) -> result/1

== system TST_InjCrv_PoI2AddCor/simulationInput/testSignals_R001 ==
  BC : BusCreator  Inputs=16
  spec_InjCrv_facPoI2Bas_mp : FromWorkspace  VariableName=testSig_InjCrv_facPoI2Bas_mp  Interpolate=off  OutputAfterFinalValue=Holding final value
  spec_InjCrv_facPoI2EffSet : FromWorkspace  VariableName=testSig_InjCrv_facPoI2EffSet  Interpolate=off  OutputAfterFinalValue=Holding final value
  spec_InjCrv_phiPoI2Bas_mp : FromWorkspace  VariableName=testSig_InjCrv_phiPoI2Bas_mp  Interpolate=off  OutputAfterFinalValue=Holding final value
  spec_InjCrv_phiPoI2Cor : FromWorkspace  VariableName=testSig_InjCrv_phiPoI2Cor  Interpolate=off  OutputAfterFinalValue=Holding final value
  spec_InjCrv_phiPoI2MaxEOMX_mp : FromWorkspace  VariableName=testSig_InjCrv_phiPoI2MaxEOMX_mp  Interpolate=off  OutputAfterFinalValue=Holding final value
  spec_InjCrv_phiPoI2Set_mp : FromWorkspace  VariableName=testSig_InjCrv_phiPoI2Set_mp  Interpolate=off  OutputAfterFinalValue=Holding final value
  spec_InjCrv_qMI1BalPoI2 : FromWorkspace  VariableName=testSig_InjCrv_qMI1BalPoI2  Interpolate=off  OutputAfterFinalValue=Holding final value
  spec_InjCrv_qPoI2Bas_mp : FromWorkspace  VariableName=testSig_InjCrv_qPoI2Bas_mp  Interpolate=off  OutputAfterFinalValue=Holding final value
  spec_InjCrv_qPoI2Cor : FromWorkspace  VariableName=testSig_InjCrv_qPoI2Cor  Interpolate=off  OutputAfterFinalValue=Holding final value
  spec_InjCrv_qPoI2Des : FromWorkspace  VariableName=testSig_InjCrv_qPoI2Des  Interpolate=off  OutputAfterFinalValue=Holding final value
  spec_InjCrv_qPoI2OfsUnLim : FromWorkspace  VariableName=testSig_InjCrv_qPoI2OfsUnLim  Interpolate=off  OutputAfterFinalValue=Holding final value
  spec_InjCrv_stShutOffPiIPoI : FromWorkspace  VariableName=testSig_InjCrv_stShutOffPiIPoI  Interpolate=off  OutputAfterFinalValue=Holding final value
  spec_InjCrv_stShutOffPoI : FromWorkspace  VariableName=testSig_InjCrv_stShutOffPoI  Interpolate=off  OutputAfterFinalValue=Holding final value
  spec_InjCrv_tiPoI2Bas_mp : FromWorkspace  VariableName=testSig_InjCrv_tiPoI2Bas_mp  Interpolate=off  OutputAfterFinalValue=Holding final value
  spec_InjCrv_tiPoI2Cor : FromWorkspace  VariableName=testSig_InjCrv_tiPoI2Cor  Interpolate=off  OutputAfterFinalValue=Holding final value
  spec_InjCrv_tiPoI2Set_mp : FromWorkspace  VariableName=testSig_InjCrv_tiPoI2Set_mp  Interpolate=off  OutputAfterFinalValue=Holding final value
  testSignals : Outport
  wires:
  BC/1 -> testSignals/1
  spec_InjCrv_qPoI2Bas_mp/1 -> BC/1  "testSig_InjCrv_qPoI2Bas_mp"
  spec_InjCrv_facPoI2Bas_mp/1 -> BC/2  "testSig_InjCrv_facPoI2Bas_mp"
  spec_InjCrv_tiPoI2Bas_mp/1 -> BC/3  "testSig_InjCrv_tiPoI2Bas_mp"
  spec_InjCrv_phiPoI2Bas_mp/1 -> BC/4  "testSig_InjCrv_phiPoI2Bas_mp"
  spec_InjCrv_qPoI2Cor/1 -> BC/5  "testSig_InjCrv_qPoI2Cor"
  spec_InjCrv_phiPoI2Cor/1 -> BC/6  "testSig_InjCrv_phiPoI2Cor"
  spec_InjCrv_tiPoI2Cor/1 -> BC/7  "testSig_InjCrv_tiPoI2Cor"
  spec_InjCrv_phiPoI2MaxEOMX_mp/1 -> BC/8  "testSig_InjCrv_phiPoI2MaxEOMX_mp"
  spec_InjCrv_stShutOffPiIPoI/1 -> BC/9  "testSig_InjCrv_stShutOffPiIPoI"
  spec_InjCrv_stShutOffPoI/1 -> BC/10  "testSig_InjCrv_stShutOffPoI"
  spec_InjCrv_qMI1BalPoI2/1 -> BC/11  "testSig_InjCrv_qMI1BalPoI2"
  spec_InjCrv_qPoI2OfsUnLim/1 -> BC/12  "testSig_InjCrv_qPoI2OfsUnLim"
  spec_InjCrv_facPoI2EffSet/1 -> BC/13  "testSig_InjCrv_facPoI2EffSet"
  spec_InjCrv_phiPoI2Set_mp/1 -> BC/14  "testSig_InjCrv_phiPoI2Set_mp"
  spec_InjCrv_tiPoI2Set_mp/1 -> BC/15  "testSig_InjCrv_tiPoI2Set_mp"
  spec_InjCrv_qPoI2Des/1 -> BC/16  "testSig_InjCrv_qPoI2Des"

== system TST_InjCrv_PoI2AddCor/simulationInput/testSignals_R002 ==
  BC : BusCreator  Inputs=16
  spec_InjCrv_facPoI2Bas_mp : FromWorkspace  VariableName=testSig_InjCrv_facPoI2Bas_mp  Interpolate=off  OutputAfterFinalValue=Holding final value
  spec_InjCrv_facPoI2EffSet : FromWorkspace  VariableName=testSig_InjCrv_facPoI2EffSet  Interpolate=off  OutputAfterFinalValue=Holding final value
  spec_InjCrv_phiPoI2Bas_mp : FromWorkspace  VariableName=testSig_InjCrv_phiPoI2Bas_mp  Interpolate=off  OutputAfterFinalValue=Holding final value
  spec_InjCrv_phiPoI2Cor : FromWorkspace  VariableName=testSig_InjCrv_phiPoI2Cor  Interpolate=off  OutputAfterFinalValue=Holding final value
  spec_InjCrv_phiPoI2MaxEOMX_mp : FromWorkspace  VariableName=testSig_InjCrv_phiPoI2MaxEOMX_mp  Interpolate=off  OutputAfterFinalValue=Holding final value
  spec_InjCrv_phiPoI2Set_mp : FromWorkspace  VariableName=testSig_InjCrv_phiPoI2Set_mp  Interpolate=off  OutputAfterFinalValue=Holding final value
  spec_InjCrv_qMI1BalPoI2 : FromWorkspace  VariableName=testSig_InjCrv_qMI1BalPoI2  Interpolate=off  OutputAfterFinalValue=Holding final value
  spec_InjCrv_qPoI2Bas_mp : FromWorkspace  VariableName=testSig_InjCrv_qPoI2Bas_mp  Interpolate=off  OutputAfterFinalValue=Holding final value
  spec_InjCrv_qPoI2Cor : FromWorkspace  VariableName=testSig_InjCrv_qPoI2Cor  Interpolate=off  OutputAfterFinalValue=Holding final value
  spec_InjCrv_qPoI2Des : FromWorkspace  VariableName=testSig_InjCrv_qPoI2Des  Interpolate=off  OutputAfterFinalValue=Holding final value
  spec_InjCrv_qPoI2OfsUnLim : FromWorkspace  VariableName=testSig_InjCrv_qPoI2OfsUnLim  Interpolate=off  OutputAfterFinalValue=Holding final value
  spec_InjCrv_stShutOffPiIPoI : FromWorkspace  VariableName=testSig_InjCrv_stShutOffPiIPoI  Interpolate=off  OutputAfterFinalValue=Holding final value
  spec_InjCrv_stShutOffPoI : FromWorkspace  VariableName=testSig_InjCrv_stShutOffPoI  Interpolate=off  OutputAfterFinalValue=Holding final value
  spec_InjCrv_tiPoI2Bas_mp : FromWorkspace  VariableName=testSig_InjCrv_tiPoI2Bas_mp  Interpolate=off  OutputAfterFinalValue=Holding final value
  spec_InjCrv_tiPoI2Cor : FromWorkspace  VariableName=testSig_InjCrv_tiPoI2Cor  Interpolate=off  OutputAfterFinalValue=Holding final value
  spec_InjCrv_tiPoI2Set_mp : FromWorkspace  VariableName=testSig_InjCrv_tiPoI2Set_mp  Interpolate=off  OutputAfterFinalValue=Holding final value
  testSignals : Outport
  wires:
  BC/1 -> testSignals/1
  spec_InjCrv_qPoI2Bas_mp/1 -> BC/1  "testSig_InjCrv_qPoI2Bas_mp"
  spec_InjCrv_facPoI2Bas_mp/1 -> BC/2  "testSig_InjCrv_facPoI2Bas_mp"
  spec_InjCrv_tiPoI2Bas_mp/1 -> BC/3  "testSig_InjCrv_tiPoI2Bas_mp"
  spec_InjCrv_phiPoI2Bas_mp/1 -> BC/4  "testSig_InjCrv_phiPoI2Bas_mp"
  spec_InjCrv_qPoI2Cor/1 -> BC/5  "testSig_InjCrv_qPoI2Cor"
  spec_InjCrv_phiPoI2Cor/1 -> BC/6  "testSig_InjCrv_phiPoI2Cor"
  spec_InjCrv_tiPoI2Cor/1 -> BC/7  "testSig_InjCrv_tiPoI2Cor"
  spec_InjCrv_phiPoI2MaxEOMX_mp/1 -> BC/8  "testSig_InjCrv_phiPoI2MaxEOMX_mp"
  spec_InjCrv_stShutOffPiIPoI/1 -> BC/9  "testSig_InjCrv_stShutOffPiIPoI"
  spec_InjCrv_stShutOffPoI/1 -> BC/10  "testSig_InjCrv_stShutOffPoI"
  spec_InjCrv_qMI1BalPoI2/1 -> BC/11  "testSig_InjCrv_qMI1BalPoI2"
  spec_InjCrv_qPoI2OfsUnLim/1 -> BC/12  "testSig_InjCrv_qPoI2OfsUnLim"
  spec_InjCrv_facPoI2EffSet/1 -> BC/13  "testSig_InjCrv_facPoI2EffSet"
  spec_InjCrv_phiPoI2Set_mp/1 -> BC/14  "testSig_InjCrv_phiPoI2Set_mp"
  spec_InjCrv_tiPoI2Set_mp/1 -> BC/15  "testSig_InjCrv_tiPoI2Set_mp"
  spec_InjCrv_qPoI2Des/1 -> BC/16  "testSig_InjCrv_qPoI2Des"

== system TST_InjCrv_PoI2AddCor/simulationInput/testSignals_R003 ==
  BC : BusCreator  Inputs=16
  spec_InjCrv_facPoI2Bas_mp : FromWorkspace  VariableName=testSig_InjCrv_facPoI2Bas_mp  Interpolate=off  OutputAfterFinalValue=Holding final value
  spec_InjCrv_facPoI2EffSet : FromWorkspace  VariableName=testSig_InjCrv_facPoI2EffSet  Interpolate=off  OutputAfterFinalValue=Holding final value
  spec_InjCrv_phiPoI2Bas_mp : FromWorkspace  VariableName=testSig_InjCrv_phiPoI2Bas_mp  Interpolate=off  OutputAfterFinalValue=Holding final value
  spec_InjCrv_phiPoI2Cor : FromWorkspace  VariableName=testSig_InjCrv_phiPoI2Cor  Interpolate=off  OutputAfterFinalValue=Holding final value
  spec_InjCrv_phiPoI2MaxEOMX_mp : FromWorkspace  VariableName=testSig_InjCrv_phiPoI2MaxEOMX_mp  Interpolate=off  OutputAfterFinalValue=Holding final value
  spec_InjCrv_phiPoI2Set_mp : FromWorkspace  VariableName=testSig_InjCrv_phiPoI2Set_mp  Interpolate=off  OutputAfterFinalValue=Holding final value
  spec_InjCrv_qMI1BalPoI2 : FromWorkspace  VariableName=testSig_InjCrv_qMI1BalPoI2  Interpolate=off  OutputAfterFinalValue=Holding final value
  spec_InjCrv_qPoI2Bas_mp : FromWorkspace  VariableName=testSig_InjCrv_qPoI2Bas_mp  Interpolate=off  OutputAfterFinalValue=Holding final value
  spec_InjCrv_qPoI2Cor : FromWorkspace  VariableName=testSig_InjCrv_qPoI2Cor  Interpolate=off  OutputAfterFinalValue=Holding final value
  spec_InjCrv_qPoI2Des : FromWorkspace  VariableName=testSig_InjCrv_qPoI2Des  Interpolate=off  OutputAfterFinalValue=Holding final value
  spec_InjCrv_qPoI2OfsUnLim : FromWorkspace  VariableName=testSig_InjCrv_qPoI2OfsUnLim  Interpolate=off  OutputAfterFinalValue=Holding final value
  spec_InjCrv_stShutOffPiIPoI : FromWorkspace  VariableName=testSig_InjCrv_stShutOffPiIPoI  Interpolate=off  OutputAfterFinalValue=Holding final value
  spec_InjCrv_stShutOffPoI : FromWorkspace  VariableName=testSig_InjCrv_stShutOffPoI  Interpolate=off  OutputAfterFinalValue=Holding final value
  spec_InjCrv_tiPoI2Bas_mp : FromWorkspace  VariableName=testSig_InjCrv_tiPoI2Bas_mp  Interpolate=off  OutputAfterFinalValue=Holding final value
  spec_InjCrv_tiPoI2Cor : FromWorkspace  VariableName=testSig_InjCrv_tiPoI2Cor  Interpolate=off  OutputAfterFinalValue=Holding final value
  spec_InjCrv_tiPoI2Set_mp : FromWorkspace  VariableName=testSig_InjCrv_tiPoI2Set_mp  Interpolate=off  OutputAfterFinalValue=Holding final value
  testSignals : Outport
  wires:
  BC/1 -> testSignals/1
  spec_InjCrv_qPoI2Bas_mp/1 -> BC/1  "testSig_InjCrv_qPoI2Bas_mp"
  spec_InjCrv_facPoI2Bas_mp/1 -> BC/2  "testSig_InjCrv_facPoI2Bas_mp"
  spec_InjCrv_tiPoI2Bas_mp/1 -> BC/3  "testSig_InjCrv_tiPoI2Bas_mp"
  spec_InjCrv_phiPoI2Bas_mp/1 -> BC/4  "testSig_InjCrv_phiPoI2Bas_mp"
  spec_InjCrv_qPoI2Cor/1 -> BC/5  "testSig_InjCrv_qPoI2Cor"
  spec_InjCrv_phiPoI2Cor/1 -> BC/6  "testSig_InjCrv_phiPoI2Cor"
  spec_InjCrv_tiPoI2Cor/1 -> BC/7  "testSig_InjCrv_tiPoI2Cor"
  spec_InjCrv_phiPoI2MaxEOMX_mp/1 -> BC/8  "testSig_InjCrv_phiPoI2MaxEOMX_mp"
  spec_InjCrv_stShutOffPiIPoI/1 -> BC/9  "testSig_InjCrv_stShutOffPiIPoI"
  spec_InjCrv_stShutOffPoI/1 -> BC/10  "testSig_InjCrv_stShutOffPoI"
  spec_InjCrv_qMI1BalPoI2/1 -> BC/11  "testSig_InjCrv_qMI1BalPoI2"
  spec_InjCrv_qPoI2OfsUnLim/1 -> BC/12  "testSig_InjCrv_qPoI2OfsUnLim"
  spec_InjCrv_facPoI2EffSet/1 -> BC/13  "testSig_InjCrv_facPoI2EffSet"
  spec_InjCrv_phiPoI2Set_mp/1 -> BC/14  "testSig_InjCrv_phiPoI2Set_mp"
  spec_InjCrv_tiPoI2Set_mp/1 -> BC/15  "testSig_InjCrv_tiPoI2Set_mp"
  spec_InjCrv_qPoI2Des/1 -> BC/16  "testSig_InjCrv_qPoI2Des"

== system TST_InjCrv_PoI2AddCor/simulationInput/testSignals_R004 ==
  BC : BusCreator  Inputs=16
  spec_InjCrv_facPoI2Bas_mp : FromWorkspace  VariableName=testSig_InjCrv_facPoI2Bas_mp  Interpolate=off  OutputAfterFinalValue=Holding final value
  spec_InjCrv_facPoI2EffSet : FromWorkspace  VariableName=testSig_InjCrv_facPoI2EffSet  Interpolate=off  OutputAfterFinalValue=Holding final value
  spec_InjCrv_phiPoI2Bas_mp : FromWorkspace  VariableName=testSig_InjCrv_phiPoI2Bas_mp  Interpolate=off  OutputAfterFinalValue=Holding final value
  spec_InjCrv_phiPoI2Cor : FromWorkspace  VariableName=testSig_InjCrv_phiPoI2Cor  Interpolate=off  OutputAfterFinalValue=Holding final value
  spec_InjCrv_phiPoI2MaxEOMX_mp : FromWorkspace  VariableName=testSig_InjCrv_phiPoI2MaxEOMX_mp  Interpolate=off  OutputAfterFinalValue=Holding final value
  spec_InjCrv_phiPoI2Set_mp : FromWorkspace  VariableName=testSig_InjCrv_phiPoI2Set_mp  Interpolate=off  OutputAfterFinalValue=Holding final value
  spec_InjCrv_qMI1BalPoI2 : FromWorkspace  VariableName=testSig_InjCrv_qMI1BalPoI2  Interpolate=off  OutputAfterFinalValue=Holding final value
  spec_InjCrv_qPoI2Bas_mp : FromWorkspace  VariableName=testSig_InjCrv_qPoI2Bas_mp  Interpolate=off  OutputAfterFinalValue=Holding final value
  spec_InjCrv_qPoI2Cor : FromWorkspace  VariableName=testSig_InjCrv_qPoI2Cor  Interpolate=off  OutputAfterFinalValue=Holding final value
  spec_InjCrv_qPoI2Des : FromWorkspace  VariableName=testSig_InjCrv_qPoI2Des  Interpolate=off  OutputAfterFinalValue=Holding final value
  spec_InjCrv_qPoI2OfsUnLim : FromWorkspace  VariableName=testSig_InjCrv_qPoI2OfsUnLim  Interpolate=off  OutputAfterFinalValue=Holding final value
  spec_InjCrv_stShutOffPiIPoI : FromWorkspace  VariableName=testSig_InjCrv_stShutOffPiIPoI  Interpolate=off  OutputAfterFinalValue=Holding final value
  spec_InjCrv_stShutOffPoI : FromWorkspace  VariableName=testSig_InjCrv_stShutOffPoI  Interpolate=off  OutputAfterFinalValue=Holding final value
  spec_InjCrv_tiPoI2Bas_mp : FromWorkspace  VariableName=testSig_InjCrv_tiPoI2Bas_mp  Interpolate=off  OutputAfterFinalValue=Holding final value
  spec_InjCrv_tiPoI2Cor : FromWorkspace  VariableName=testSig_InjCrv_tiPoI2Cor  Interpolate=off  OutputAfterFinalValue=Holding final value
  spec_InjCrv_tiPoI2Set_mp : FromWorkspace  VariableName=testSig_InjCrv_tiPoI2Set_mp  Interpolate=off  OutputAfterFinalValue=Holding final value
  testSignals : Outport
  wires:
  BC/1 -> testSignals/1
  spec_InjCrv_qPoI2Bas_mp/1 -> BC/1  "testSig_InjCrv_qPoI2Bas_mp"
  spec_InjCrv_facPoI2Bas_mp/1 -> BC/2  "testSig_InjCrv_facPoI2Bas_mp"
  spec_InjCrv_tiPoI2Bas_mp/1 -> BC/3  "testSig_InjCrv_tiPoI2Bas_mp"
  spec_InjCrv_phiPoI2Bas_mp/1 -> BC/4  "testSig_InjCrv_phiPoI2Bas_mp"
  spec_InjCrv_qPoI2Cor/1 -> BC/5  "testSig_InjCrv_qPoI2Cor"
  spec_InjCrv_phiPoI2Cor/1 -> BC/6  "testSig_InjCrv_phiPoI2Cor"
  spec_InjCrv_tiPoI2Cor/1 -> BC/7  "testSig_InjCrv_tiPoI2Cor"
  spec_InjCrv_phiPoI2MaxEOMX_mp/1 -> BC/8  "testSig_InjCrv_phiPoI2MaxEOMX_mp"
  spec_InjCrv_stShutOffPiIPoI/1 -> BC/9  "testSig_InjCrv_stShutOffPiIPoI"
  spec_InjCrv_stShutOffPoI/1 -> BC/10  "testSig_InjCrv_stShutOffPoI"
  spec_InjCrv_qMI1BalPoI2/1 -> BC/11  "testSig_InjCrv_qMI1BalPoI2"
  spec_InjCrv_qPoI2OfsUnLim/1 -> BC/12  "testSig_InjCrv_qPoI2OfsUnLim"
  spec_InjCrv_facPoI2EffSet/1 -> BC/13  "testSig_InjCrv_facPoI2EffSet"
  spec_InjCrv_phiPoI2Set_mp/1 -> BC/14  "testSig_InjCrv_phiPoI2Set_mp"
  spec_InjCrv_tiPoI2Set_mp/1 -> BC/15  "testSig_InjCrv_tiPoI2Set_mp"
  spec_InjCrv_qPoI2Des/1 -> BC/16  "testSig_InjCrv_qPoI2Des"

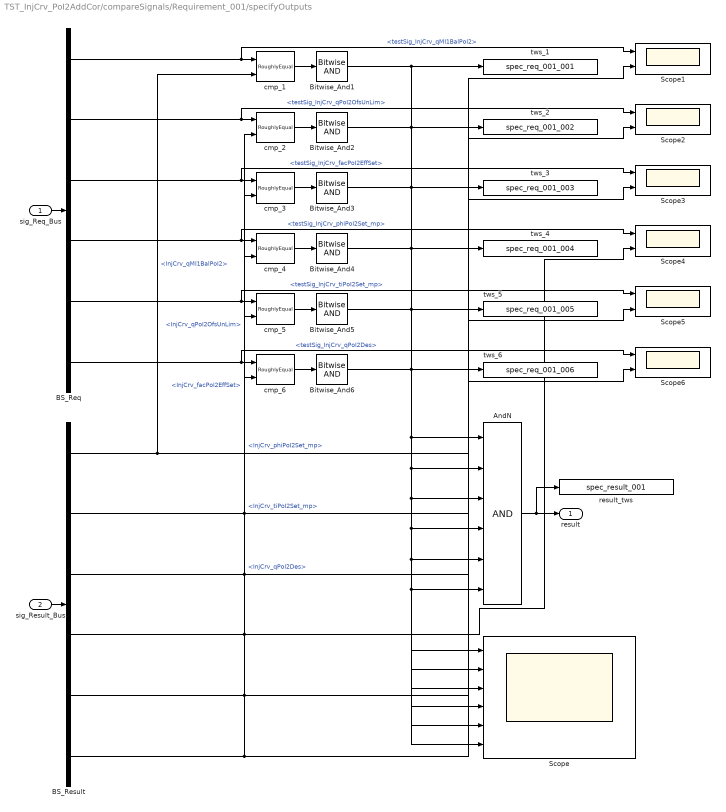
== system TST_InjCrv_PoI2AddCor/compareSignals/Requirement_001/specifyOutputs ==
  sig_Req_Bus : Inport
  sig_Result_Bus : Inport  Port=2
  AndN : Logic  Inputs=6
  BS_Req : BusSelector  OutputSignals=testSig_InjCrv_qMI1BalPoI2,testSig_InjCrv_qPoI2OfsUnLim,testSig_InjCrv_facPoI2EffSet,testSig_InjCrv_phiPoI2Set_mp,testSig_InjCrv_tiPoI2Set_mp,testSig_InjCrv_qPoI2Des
  BS_Result : BusSelector  OutputSignals=InjCrv_qMI1BalPoI2,InjCrv_qPoI2OfsUnLim,InjCrv_facPoI2EffSet,InjCrv_phiPoI2Set_mp,InjCrv_tiPoI2Set_mp,InjCrv_qPoI2Des
  Bitwise_And{1..6} (6 alike) : simulink/Logic and Bit Operations/Bitwise Operator  logicop=AND  UseBitMask=off  BitMask=bin2dec('11011001')  BitMaskRealWorld=Stored Integer
  Scope : Scope  NumInputPorts=6
  Scope{1..6} (6 alike) : Scope  NumInputPorts=2
  cmp_{1..4,6} (5 alike) : UnitTest_Lib/RoughlyEqual  slope=0.1
  cmp_5 : UnitTest_Lib/RoughlyEqual  slope=1
  result_tws : ToWorkspace  VariableName=spec_result_001
  tws_1 : ToWorkspace  VariableName=spec_req_001_001
  tws_2 : ToWorkspace  VariableName=spec_req_001_002
  tws_3 : ToWorkspace  VariableName=spec_req_001_003
  tws_4 : ToWorkspace  VariableName=spec_req_001_004
  tws_5 : ToWorkspace  VariableName=spec_req_001_005
  tws_6 : ToWorkspace  VariableName=spec_req_001_006
  result : Outport
  wires:
  sig_Req_Bus/1 -> BS_Req/1
  sig_Result_Bus/1 -> BS_Result/1
  AndN/1 -> result/1, result_tws/1
  BS_Req/1 -> cmp_1/1, Scope1/1  "<testSig_InjCrv_qMI1BalPoI2>"
  BS_Result/1 -> cmp_1/2, Scope1/2  "<InjCrv_qMI1BalPoI2>"
  cmp_1/1 -> Bitwise_And1/1
  Bitwise_And1/1 -> AndN/1, Scope/1, tws_1/1
  BS_Req/2 -> cmp_2/1, Scope2/1  "<testSig_InjCrv_qPoI2OfsUnLim>"
  BS_Result/2 -> cmp_2/2, Scope2/2  "<InjCrv_qPoI2OfsUnLim>"
  cmp_2/1 -> Bitwise_And2/1
  Bitwise_And2/1 -> AndN/2, Scope/2, tws_2/1
  BS_Req/3 -> cmp_3/1, Scope3/1  "<testSig_InjCrv_facPoI2EffSet>"
  BS_Result/3 -> cmp_3/2, Scope3/2  "<InjCrv_facPoI2EffSet>"
  cmp_3/1 -> Bitwise_And3/1
  Bitwise_And3/1 -> AndN/3, Scope/3, tws_3/1
  BS_Req/4 -> cmp_4/1, Scope4/1  "<testSig_InjCrv_phiPoI2Set_mp>"
  BS_Result/4 -> cmp_4/2, Scope4/2  "<InjCrv_phiPoI2Set_mp>"
  cmp_4/1 -> Bitwise_And4/1
  Bitwise_And4/1 -> AndN/4, Scope/4, tws_4/1
  BS_Req/5 -> cmp_5/1, Scope5/1  "<testSig_InjCrv_tiPoI2Set_mp>"
  BS_Result/5 -> cmp_5/2, Scope5/2  "<InjCrv_tiPoI2Set_mp>"
  cmp_5/1 -> Bitwise_And5/1
  Bitwise_And5/1 -> AndN/5, Scope/5, tws_5/1
  BS_Req/6 -> cmp_6/1, Scope6/1  "<testSig_InjCrv_qPoI2Des>"
  BS_Result/6 -> cmp_6/2, Scope6/2  "<InjCrv_qPoI2Des>"
  cmp_6/1 -> Bitwise_And6/1
  Bitwise_And6/1 -> AndN/6, Scope/6, tws_6/1

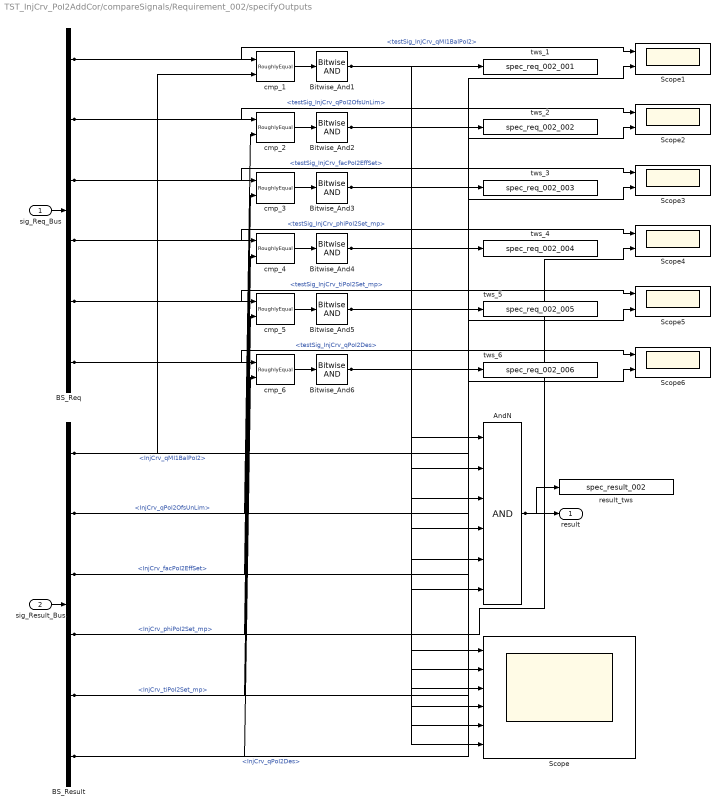
== system TST_InjCrv_PoI2AddCor/compareSignals/Requirement_002/specifyOutputs ==
  sig_Req_Bus : Inport
  sig_Result_Bus : Inport  Port=2
  AndN : Logic  Inputs=6
  BS_Req : BusSelector  OutputSignals=testSig_InjCrv_qMI1BalPoI2,testSig_InjCrv_qPoI2OfsUnLim,testSig_InjCrv_facPoI2EffSet,testSig_InjCrv_phiPoI2Set_mp,testSig_InjCrv_tiPoI2Set_mp,testSig_InjCrv_qPoI2Des
  BS_Result : BusSelector  OutputSignals=InjCrv_qMI1BalPoI2,InjCrv_qPoI2OfsUnLim,InjCrv_facPoI2EffSet,InjCrv_phiPoI2Set_mp,InjCrv_tiPoI2Set_mp,InjCrv_qPoI2Des
  Bitwise_And{1..6} (6 alike) : simulink/Logic and Bit Operations/Bitwise Operator  logicop=AND  UseBitMask=off  BitMask=bin2dec('11011001')  BitMaskRealWorld=Stored Integer
  Scope : Scope  NumInputPorts=6
  Scope{1..6} (6 alike) : Scope  NumInputPorts=2
  cmp_{1..6} (6 alike) : UnitTest_Lib/RoughlyEqual  slope=0.1
  result_tws : ToWorkspace  VariableName=spec_result_002
  tws_1 : ToWorkspace  VariableName=spec_req_002_001
  tws_2 : ToWorkspace  VariableName=spec_req_002_002
  tws_3 : ToWorkspace  VariableName=spec_req_002_003
  tws_4 : ToWorkspace  VariableName=spec_req_002_004
  tws_5 : ToWorkspace  VariableName=spec_req_002_005
  tws_6 : ToWorkspace  VariableName=spec_req_002_006
  result : Outport
  wires:
  sig_Req_Bus/1 -> BS_Req/1
  sig_Result_Bus/1 -> BS_Result/1
  AndN/1 -> result/1, result_tws/1
  BS_Req/1 -> cmp_1/1, Scope1/1  "<testSig_InjCrv_qMI1BalPoI2>"
  BS_Result/1 -> cmp_1/2, Scope1/2  "<InjCrv_qMI1BalPoI2>"
  cmp_1/1 -> Bitwise_And1/1
  Bitwise_And1/1 -> tws_1/1, AndN/1, Scope/1
  BS_Req/2 -> cmp_2/1, Scope2/1  "<testSig_InjCrv_qPoI2OfsUnLim>"
  BS_Result/2 -> cmp_2/2, Scope2/2  "<InjCrv_qPoI2OfsUnLim>"
  cmp_2/1 -> Bitwise_And2/1
  Bitwise_And2/1 -> tws_2/1, AndN/2, Scope/2
  BS_Req/3 -> cmp_3/1, Scope3/1  "<testSig_InjCrv_facPoI2EffSet>"
  BS_Result/3 -> cmp_3/2, Scope3/2  "<InjCrv_facPoI2EffSet>"
  cmp_3/1 -> Bitwise_And3/1
  Bitwise_And3/1 -> tws_3/1, AndN/3, Scope/3
  BS_Req/4 -> cmp_4/1, Scope4/1  "<testSig_InjCrv_phiPoI2Set_mp>"
  BS_Result/4 -> cmp_4/2, Scope4/2  "<InjCrv_phiPoI2Set_mp>"
  cmp_4/1 -> Bitwise_And4/1
  Bitwise_And4/1 -> tws_4/1, AndN/4, Scope/4
  BS_Req/5 -> cmp_5/1, Scope5/1  "<testSig_InjCrv_tiPoI2Set_mp>"
  BS_Result/5 -> cmp_5/2, Scope5/2  "<InjCrv_tiPoI2Set_mp>"
  cmp_5/1 -> Bitwise_And5/1
  Bitwise_And5/1 -> tws_5/1, AndN/5, Scope/5
  BS_Req/6 -> cmp_6/1, Scope6/1  "<testSig_InjCrv_qPoI2Des>"
  BS_Result/6 -> cmp_6/2, Scope6/2  "<InjCrv_qPoI2Des>"
  cmp_6/1 -> Bitwise_And6/1
  Bitwise_And6/1 -> tws_6/1, AndN/6, Scope/6

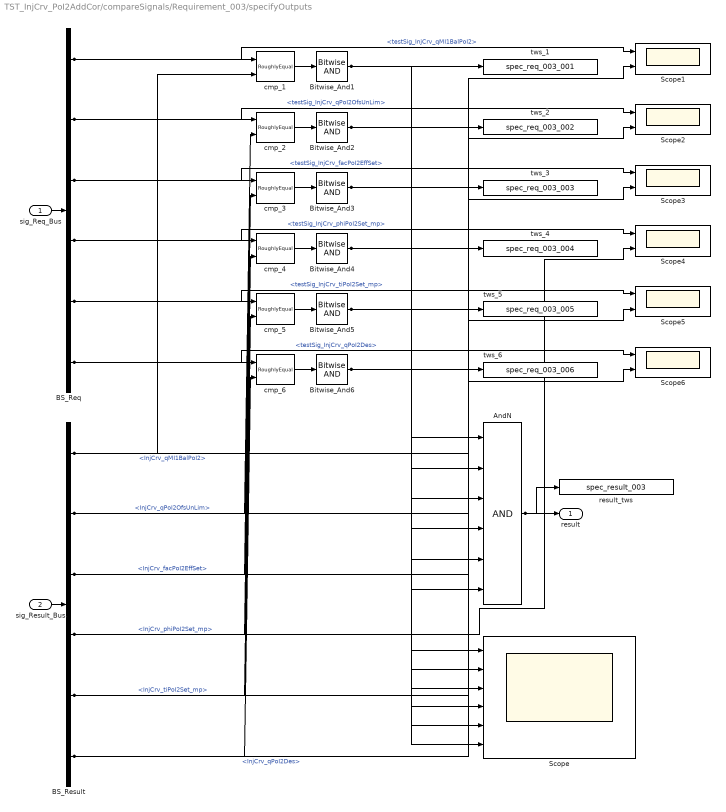
== system TST_InjCrv_PoI2AddCor/compareSignals/Requirement_003/specifyOutputs ==
  sig_Req_Bus : Inport
  sig_Result_Bus : Inport  Port=2
  AndN : Logic  Inputs=6
  BS_Req : BusSelector  OutputSignals=testSig_InjCrv_qMI1BalPoI2,testSig_InjCrv_qPoI2OfsUnLim,testSig_InjCrv_facPoI2EffSet,testSig_InjCrv_phiPoI2Set_mp,testSig_InjCrv_tiPoI2Set_mp,testSig_InjCrv_qPoI2Des
  BS_Result : BusSelector  OutputSignals=InjCrv_qMI1BalPoI2,InjCrv_qPoI2OfsUnLim,InjCrv_facPoI2EffSet,InjCrv_phiPoI2Set_mp,InjCrv_tiPoI2Set_mp,InjCrv_qPoI2Des
  Bitwise_And{1..6} (6 alike) : simulink/Logic and Bit Operations/Bitwise Operator  logicop=AND  UseBitMask=off  BitMask=bin2dec('11011001')  BitMaskRealWorld=Stored Integer
  Scope : Scope  NumInputPorts=6
  Scope{1..6} (6 alike) : Scope  NumInputPorts=2
  cmp_{1..6} (6 alike) : UnitTest_Lib/RoughlyEqual  slope=0.1
  result_tws : ToWorkspace  VariableName=spec_result_003
  tws_1 : ToWorkspace  VariableName=spec_req_003_001
  tws_2 : ToWorkspace  VariableName=spec_req_003_002
  tws_3 : ToWorkspace  VariableName=spec_req_003_003
  tws_4 : ToWorkspace  VariableName=spec_req_003_004
  tws_5 : ToWorkspace  VariableName=spec_req_003_005
  tws_6 : ToWorkspace  VariableName=spec_req_003_006
  result : Outport
  wires:
  sig_Req_Bus/1 -> BS_Req/1
  sig_Result_Bus/1 -> BS_Result/1
  AndN/1 -> result/1, result_tws/1
  BS_Req/1 -> cmp_1/1, Scope1/1  "<testSig_InjCrv_qMI1BalPoI2>"
  BS_Result/1 -> cmp_1/2, Scope1/2  "<InjCrv_qMI1BalPoI2>"
  cmp_1/1 -> Bitwise_And1/1
  Bitwise_And1/1 -> tws_1/1, AndN/1, Scope/1
  BS_Req/2 -> cmp_2/1, Scope2/1  "<testSig_InjCrv_qPoI2OfsUnLim>"
  BS_Result/2 -> cmp_2/2, Scope2/2  "<InjCrv_qPoI2OfsUnLim>"
  cmp_2/1 -> Bitwise_And2/1
  Bitwise_And2/1 -> tws_2/1, AndN/2, Scope/2
  BS_Req/3 -> cmp_3/1, Scope3/1  "<testSig_InjCrv_facPoI2EffSet>"
  BS_Result/3 -> cmp_3/2, Scope3/2  "<InjCrv_facPoI2EffSet>"
  cmp_3/1 -> Bitwise_And3/1
  Bitwise_And3/1 -> tws_3/1, AndN/3, Scope/3
  BS_Req/4 -> cmp_4/1, Scope4/1  "<testSig_InjCrv_phiPoI2Set_mp>"
  BS_Result/4 -> cmp_4/2, Scope4/2  "<InjCrv_phiPoI2Set_mp>"
  cmp_4/1 -> Bitwise_And4/1
  Bitwise_And4/1 -> tws_4/1, AndN/4, Scope/4
  BS_Req/5 -> cmp_5/1, Scope5/1  "<testSig_InjCrv_tiPoI2Set_mp>"
  BS_Result/5 -> cmp_5/2, Scope5/2  "<InjCrv_tiPoI2Set_mp>"
  cmp_5/1 -> Bitwise_And5/1
  Bitwise_And5/1 -> tws_5/1, AndN/5, Scope/5
  BS_Req/6 -> cmp_6/1, Scope6/1  "<testSig_InjCrv_qPoI2Des>"
  BS_Result/6 -> cmp_6/2, Scope6/2  "<InjCrv_qPoI2Des>"
  cmp_6/1 -> Bitwise_And6/1
  Bitwise_And6/1 -> tws_6/1, AndN/6, Scope/6
